simulink model "bTestModel"  (R2015b)
settings: Solver=ode45  StartTime=0.0  StopTime=12  RelTol=1e-6
undefined symbols (not defined in the file): B_f, g, J_f, l_f, l_w, m_f, m_w
settings Model: Creator=USUARIO  LastModifiedBy=USUARIO
settings DataIOCC: LimitDataPoints=off  SaveFormat=Array
settings DebuggingCC: SolverPrmCheckMsg=warning
settings HardwareCC: ProdBitPerPointer=32  ProdLargestAtomicFloat=None  ProdIntDivRoundTo=Undefined  ProdEndianess=Unspecified  ProdWordSize=32  ProdHWDeviceType=32-bit Generic
settings GRTTargetCC: GeneratePreprocessorConditionals=Disable all
settings ConfigComp: CovModelRefEnable=Off  CovSFcnEnable=off

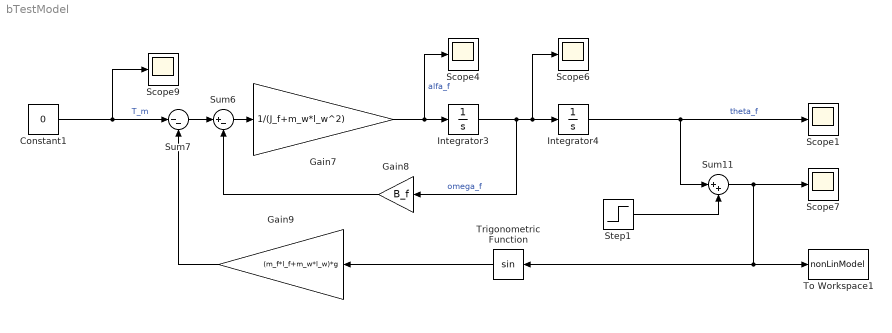
== system bTestModel ==
  Constant1 : Constant  Value=0
  Gain7 : Gain  Gain=1/(J_f+m_w*l_w^2)
  Gain8 : Gain  Gain=B_f
  Gain9 : Gain  Gain=(m_f*l_f+m_w*l_w)*g
  Integrator3 : Integrator
  Integrator4 : Integrator
  Scope{1,4,6..7,9} (5 alike) : Scope
  Step1 : Step  Time=0  After=-pi/4  SampleTime=0
  Sum11 : Sum  Inputs=|++
  Sum6 : Sum  Inputs=|+-
  Sum7 : Sum  Inputs=|--
  To Workspace1 : ToWorkspace  VariableName=nonLinModel  SaveFormat=Timeseries  SampleTime=-1
  Trigonometric Function : Trigonometry
  wires:
  Gain7/1 -> Scope4/1, Integrator3/1  "alfa_f"
  Integrator3/1 -> Gain8/1, Scope6/1, Integrator4/1  "omega_f"
  Sum6/1 -> Gain7/1
  Sum7/1 -> Sum6/1
  Gain8/1 -> Sum6/2
  Gain9/1 -> Sum7/2
  Constant1/1 -> Sum7/1, Scope9/1  "T_m"
  Integrator4/1 -> Scope1/1, Sum11/1  "theta_f"
  Step1/1 -> Sum11/2
  Sum11/1 -> Scope7/1, Trigonometric Function/1, To Workspace1/1
  Trigonometric Function/1 -> Gain9/1
